simulink model "f_pack"  (R2016b)
settings: Solver=FixedStepDiscrete  StartTime=0.0  StopTime=800000  RelTol=1e-3
undefined symbols (not defined in the file): fft_stages
libraries: xbsIndex_r4 x729, simulink x1, casper_library_misc x1
(part 1 of 6)
settings Model: Creator=andrew  LastModifiedBy=andrew
settings DataIOCC: LimitDataPoints=on  SaveFormat=Array
settings OptimizationCC: ExpressionDepthLimit=2147483647  LifeSpan=inf
settings DebuggingCC: UnderspecifiedInitializationDetection=Classic  MergeDetectMultiDrivingBlocksExec=none  SolverPrmCheckMsg=warning  StateNameClashWarn=warning  SFUnexpectedBacktrackingDiag=warning  SFNoUnconditionalDefaultTransitionDiag=warning  SFExecutionAtInitializationDiag=none
settings HardwareCC: ProdBitPerPointer=32  ProdBitPerSizeT=32  ProdBitPerPtrDiffT=32  ProdLargestAtomicFloat=None  ProdIntDivRoundTo=Undefined  ProdEndianess=Unspecified  ProdWordSize=32  ProdHWDeviceType=32-bit Generic
settings ModelReferenceCC: PropagateSignalLabelsOutOfModel=off
settings GRTTargetCC: TargetLangStandard=C89/C90 (ANSI)  GeneratePreprocessorConditionals=Disable all
settings ConfigComp: CovMetricSettings=dw  CovHtmlReporting=on  CovSaveCumulativeToWorkspaceVar=on  CovSaveSingleToWorkspaceVar=on  CovExternalEMLEnable=off

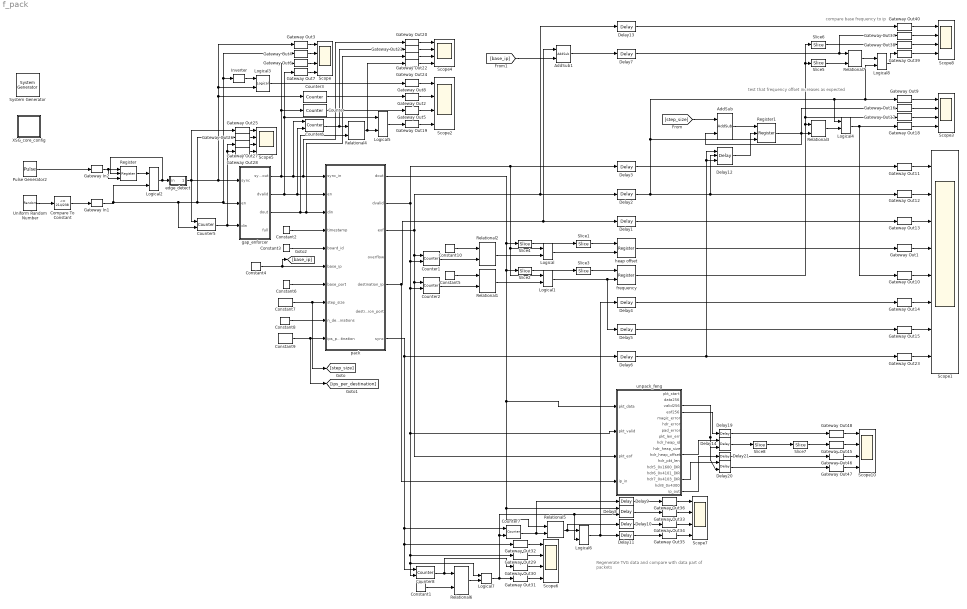
== system f_pack ==
  note: compare base frequency to ip
  note: Regenerate TVG data and compare with data part of
      | packets
  note: test that frequency offset increases as expected
  " System Generator" : xbsIndex_r4/ System Generator  Tag=genX  xilinxfamily=virtex6  part=xc6vsx475t  speed=-1  package=ff1759  synthesis_tool=XST  clock_wrapper=Clock Enables  directory=./r2_128w_32k_16x_r431/sysgen  proj_type=Project Navigator  Synth_file=XST Defaults  Impl_file=ISE Defaults  testbench=off  simulink_period=1  sysclk_period=4.3478  dcm_input_clock_period=100  incr_netlist=off  trim_vbits=Everywhere in SubSystem  dbl_ovrd=According to Block Masks  core_generation=According to Block Masks  run_coregen=off  deprecated_control=off  eval_field=0  block_type=sysgen
      settings: block_version=10.1.3
  AddSub : xbsIndex_r4/AddSub  mode=Addition  use_carryin=off  use_carryout=off  en=off  latency=0  precision=User Defined  arith_type=Unsigned  n_bits=12  bin_pt=0  quantization=Truncate  overflow=Wrap  use_behavioral_HDL=off  hw_selection=Fabric  pipelined=off  dbl_ovrd=off  block_type=addsub
  AddSub1 : xbsIndex_r4/AddSub  mode=Subtraction  use_carryin=off  use_carryout=off  en=off  latency=0  precision=Full  arith_type=Unsigned  n_bits=12  bin_pt=0  quantization=Truncate  overflow=Wrap  use_behavioral_HDL=off  hw_selection=Fabric  pipelined=off  dbl_ovrd=off  block_type=addsub
  Compare To Constant : simulink/Logic and Bit Operations/Compare To Constant  relop=<=  const=214/238  OutDataTypeStr=boolean
  Constant1 : xbsIndex_r4/Constant  const=2  gui_display_data_type=Fixed-point  arith_type=Unsigned  n_bits=6  bin_pt=0  preci_type=Single  exp_width=8  frac_width=24  explicit_period=on  period=1  equ=P=C  opselect=C  inp2=PCIN>>17  opr=+  inp1=P  carry=CIN  dbl_ovrd=off  block_type=constant
  Constant10 : xbsIndex_r4/Constant  const=0  gui_display_data_type=Fixed-point  arith_type=Unsigned  n_bits=10  bin_pt=0  preci_type=Single  exp_width=8  frac_width=24  explicit_period=off  period=1  equ=P=C  opselect=C  inp2=PCIN>>17  opr=+  inp1=P  carry=CIN  dbl_ovrd=off  block_type=constant
  Constant2 : xbsIndex_r4/Constant  const=0  gui_display_data_type=Fixed-point  arith_type=Unsigned  n_bits=48  bin_pt=0  preci_type=Single  exp_width=8  frac_width=24  explicit_period=on  period=1  equ=P=C  opselect=C  inp2=PCIN>>17  opr=+  inp1=P  carry=CIN  dbl_ovrd=off  block_type=constant
  Constant3 : xbsIndex_r4/Constant  const=0  gui_display_data_type=Fixed-point  arith_type=Unsigned  n_bits=16  bin_pt=0  preci_type=Single  exp_width=8  frac_width=24  explicit_period=on  period=1  equ=P=C  opselect=C  inp2=PCIN>>17  opr=+  inp1=P  carry=CIN  dbl_ovrd=off  block_type=constant
  Constant4 : xbsIndex_r4/Constant  const=0  gui_display_data_type=Fixed-point  arith_type=Unsigned  n_bits=32  bin_pt=0  preci_type=Single  exp_width=8  frac_width=24  explicit_period=on  period=1  equ=P=C  opselect=C  inp2=PCIN>>17  opr=+  inp1=P  carry=CIN  dbl_ovrd=off  block_type=constant
  Constant5 : xbsIndex_r4/Constant  const=1  gui_display_data_type=Fixed-point  arith_type=Unsigned  n_bits=10  bin_pt=0  preci_type=Single  exp_width=8  frac_width=24  explicit_period=off  period=1  equ=P=C  opselect=C  inp2=PCIN>>17  opr=+  inp1=P  carry=CIN  dbl_ovrd=off  block_type=constant
  Constant6 : xbsIndex_r4/Constant  const=0  gui_display_data_type=Fixed-point  arith_type=Unsigned  n_bits=16  bin_pt=0  preci_type=Single  exp_width=8  frac_width=24  explicit_period=on  period=1  equ=P=C  opselect=C  inp2=PCIN>>17  opr=+  inp1=P  carry=CIN  dbl_ovrd=off  block_type=constant
  Constant7 : xbsIndex_r4/Constant  const=256  gui_display_data_type=Fixed-point  arith_type=Unsigned  n_bits=12  bin_pt=0  preci_type=Single  exp_width=8  frac_width=24  explicit_period=on  period=1  equ=P=C  opselect=C  inp2=PCIN>>17  opr=+  inp1=P  carry=CIN  dbl_ovrd=off  block_type=constant
  Constant8 : xbsIndex_r4/Constant  const=16  gui_display_data_type=Fixed-point  arith_type=Unsigned  n_bits=9  bin_pt=0  preci_type=Single  exp_width=8  frac_width=24  explicit_period=on  period=1  equ=P=C  opselect=C  inp2=PCIN>>17  opr=+  inp1=P  carry=CIN  dbl_ovrd=off  block_type=constant
  Constant9 : xbsIndex_r4/Constant  const=1  gui_display_data_type=Fixed-point  arith_type=Unsigned  n_bits=6  bin_pt=4  preci_type=Single  exp_width=8  frac_width=24  explicit_period=on  period=1  equ=P=C  opselect=C  inp2=PCIN>>17  opr=+  inp1=P  carry=CIN  dbl_ovrd=off  block_type=constant
  Counter : xbsIndex_r4/Counter  cnt_type=Free Running  cnt_to=Inf  operation=Up  start_count=0  cnt_by_val=1  arith_type=Unsigned  n_bits=16  bin_pt=0  load_pin=off  rst=off  en=on  explicit_period=on  period=1  use_behavioral_HDL=off  implementation=Fabric  dbl_ovrd=off  block_type=counter
  Counter1 : xbsIndex_r4/Counter  cnt_type=Free Running  cnt_to=2^8+10  operation=Up  start_count=0  cnt_by_val=1  arith_type=Unsigned  n_bits=10  bin_pt=0  load_pin=off  rst=on  en=on  explicit_period=on  period=1  use_behavioral_HDL=off  implementation=Fabric  dbl_ovrd=off  block_type=counter
  Counter2 : xbsIndex_r4/Counter  cnt_type=Free Running  cnt_to=2^8+10  operation=Up  start_count=0  cnt_by_val=1  arith_type=Unsigned  n_bits=10  bin_pt=0  load_pin=off  rst=on  en=on  explicit_period=on  period=1  use_behavioral_HDL=off  implementation=Fabric  dbl_ovrd=off  block_type=counter
  Counter3 : xbsIndex_r4/Counter  cnt_type=Free Running  cnt_to=Inf  operation=Up  start_count=0  cnt_by_val=1  arith_type=Unsigned  n_bits=16  bin_pt=0  load_pin=off  rst=off  en=on  explicit_period=on  period=1  use_behavioral_HDL=off  implementation=Fabric  dbl_ovrd=off  block_type=counter
  Counter5 : xbsIndex_r4/Counter  cnt_type=Free Running  cnt_to=Inf  operation=Up  start_count=0  cnt_by_val=1  arith_type=Unsigned  n_bits=256  bin_pt=0  load_pin=off  rst=on  en=on  explicit_period=on  period=1  use_behavioral_HDL=off  implementation=Fabric  dbl_ovrd=off  block_type=counter
  Counter6 : xbsIndex_r4/Counter  cnt_type=Free Running  cnt_to=Inf  operation=Up  start_count=0  cnt_by_val=1  arith_type=Unsigned  n_bits=256  bin_pt=0  load_pin=off  rst=on  en=on  explicit_period=on  period=1  use_behavioral_HDL=off  implementation=Fabric  dbl_ovrd=off  block_type=counter
  Counter7 : xbsIndex_r4/Counter  cnt_type=Free Running  cnt_to=Inf  operation=Up  start_count=0  cnt_by_val=1  arith_type=Unsigned  n_bits=256  bin_pt=0  load_pin=off  rst=on  en=on  explicit_period=on  period=1  use_behavioral_HDL=off  implementation=Fabric  dbl_ovrd=off  block_type=counter
  Counter8 : xbsIndex_r4/Counter  cnt_type=Count Limited  cnt_to=34  operation=Up  start_count=0  cnt_by_val=1  arith_type=Unsigned  n_bits=6  bin_pt=0  load_pin=off  rst=on  en=on  explicit_period=on  period=1  use_behavioral_HDL=off  implementation=Fabric  dbl_ovrd=off  block_type=counter
  Delay{1..7,9..11,13,19,21} (13 alike) : xbsIndex_r4/Delay  rst=off  infoeditControl=Selection of Reset will increase slice count due to use of real FFs and instead of SRLs  en=off  latency=1  reg_retiming=off  dbl_ovrd=off  block_type=delay
  Delay12 : xbsIndex_r4/Delay  rst=on  infoeditControl=Selection of Reset will increase slice count due to use of real FFs and instead of SRLs  en=on  latency=1  reg_retiming=off  dbl_ovrd=off  block_type=delay
      settings: infoedit=Hardware notes: A delay line is a chain, each link of which is an SRL16 or SRL32 followed by a flip-flop.
  Delay14 : xbsIndex_r4/Delay  rst=off  infoeditControl=Selection of Reset will increase slice count due to use of real FFs and instead of SRLs  en=on  latency=1  reg_retiming=off  dbl_ovrd=off  block_type=delay
      settings: infoedit=Hardware notes: A delay line is a chain, each link of which is an SRL16 or SRL32 followed by a flip-flop.
  Delay20 : xbsIndex_r4/Delay  rst=off  infoeditControl=Selection of Reset will increase slice count due to use of real FFs and instead of SRLs  en=on  latency=1  reg_retiming=off  dbl_ovrd=off  block_type=delay
      settings: infoedit=Hardware notes: A delay line is a chain, each link of which is an SRL16 or SRL32 followed by a flip-flop.
  Delay8 : xbsIndex_r4/Delay  rst=off  infoeditControl=Selection of Reset will increase slice count due to use of real FFs and instead of SRLs  en=on  latency=1  reg_retiming=off  dbl_ovrd=off  block_type=delay
      settings: infoedit=Hardware notes: A delay line is a chain, each link of which is an SRL16 or SRL32 followed by a flip-flop.
  Gateway In1 : xbsIndex_r4/Gateway In  gui_display_data_type=Boolean  arith_type=Boolean  n_bits=16  bin_pt=14  preci_type=Single  exp_width=8  frac_width=24  rows=1  columns=1  quantization="Round  (unbiased: +/- Inf)"  overflow=Saturate  period=1  UseAsADC=off  ADCChannel='1'  interface=None  automatic_assignment=on  address_offset=hex2dec('00')  intf_name=''  intf_description=''  default_value=0  timing_constraint=None  locs_specified=off  LOCs={}  io_standard={}  inherit_from_input=off  hdl_port=on  dbl_ovrd=off  block_type=gatewayin
  Gateway In2 : xbsIndex_r4/Gateway In  gui_display_data_type=Boolean  arith_type=Boolean  n_bits=16  bin_pt=14  preci_type=Single  exp_width=8  frac_width=24  rows=1  columns=1  quantization="Round  (unbiased: +/- Inf)"  overflow=Saturate  period=1  UseAsADC=off  ADCChannel='1'  interface=None  automatic_assignment=on  address_offset=hex2dec('00')  intf_name=''  intf_description=''  default_value=0  timing_constraint=None  locs_specified=off  LOCs={}  io_standard={}  inherit_from_input=off  hdl_port=on  dbl_ovrd=off  block_type=gatewayin
  Gateway Out{1..40,45..48} (44 alike) : xbsIndex_r4/Gateway Out  inherit_from_input=off  hdl_port=on  rows=1  columns=1  UseAsDAC=off  DACChannel='1'  interface=None  automatic_assignment=on  address_offset=hex2dec('00')  intf_name=''  intf_description=''  timing_constraint=None  locs_specified=off  LOCs={}  io_standard={}  block_type=gatewayout
  Inverter : xbsIndex_r4/Inverter  en=off  latency=0  dbl_ovrd=off  block_type=inv
  Logical{,1..8} (9 alike) : xbsIndex_r4/Logical  logical_function=AND  inputs=2  en=off  latency=0  precision=Full  arith_type=Unsigned  n_bits=16  bin_pt=0  align_bp=on  dbl_ovrd=off  block_type=logical
  Pulse Generator2 : DiscretePulseGenerator  Period=2^(10+8)  PhaseDelay=2001
  Register : xbsIndex_r4/Register  init=0  rst=on  en=on  dbl_ovrd=off  block_type=register
  Register1 : xbsIndex_r4/Register  init=0  rst=on  en=on  dbl_ovrd=off  block_type=register
  Relational1 : xbsIndex_r4/Relational  mode=a=b  op_type=Bool  en=off  latency=0  dbl_ovrd=off  block_type=relational
  Relational2 : xbsIndex_r4/Relational  mode=a=b  op_type=Bool  en=off  latency=0  dbl_ovrd=off  block_type=relational
  Relational{3..5,7} (4 alike) : xbsIndex_r4/Relational  mode=a!=b  op_type=Bool  en=off  latency=0  dbl_ovrd=off  block_type=relational
  Relational6 : xbsIndex_r4/Relational  mode=a>b  op_type=Bool  en=off  latency=0  dbl_ovrd=off  block_type=relational
  Scope{,2..8,10} (9 alike) : Scope  NumInputPorts=4
  Scope1 : Scope  NumInputPorts=8
  Slice1 : xbsIndex_r4/Slice  nbits=30  boolean_output=off  mode=Two Bit Locations  bit1=0  base1=MSB of Input  bit0=10  base0=LSB of Input  dbl_ovrd=off  block_type=slice
  Slice2 : xbsIndex_r4/Slice  nbits=48  boolean_output=off  mode=Lower Bit Location + Width  bit1=0  base1=MSB of Input  bit0=0  base0=LSB of Input  dbl_ovrd=off  block_type=slice
  Slice3 : xbsIndex_r4/Slice  nbits=12  boolean_output=off  mode=Lower Bit Location + Width  bit1=0  base1=MSB of Input  bit0=0  base0=LSB of Input  dbl_ovrd=off  block_type=slice
  Slice4 : xbsIndex_r4/Slice  nbits=48  boolean_output=off  mode=Lower Bit Location + Width  bit1=0  base1=MSB of Input  bit0=0  base0=LSB of Input  dbl_ovrd=off  block_type=slice
  Slice5 : xbsIndex_r4/Slice  nbits=30  boolean_output=off  mode=Two Bit Locations  bit1=0  base1=MSB of Input  bit0=8  base0=LSB of Input  dbl_ovrd=off  block_type=slice
  Slice6 : xbsIndex_r4/Slice  nbits=30  boolean_output=off  mode=Two Bit Locations  bit1=0  base1=MSB of Input  bit0=8  base0=LSB of Input  dbl_ovrd=off  block_type=slice
  Slice7 : xbsIndex_r4/Slice  nbits=30  boolean_output=off  mode=Two Bit Locations  bit1=0  base1=MSB of Input  bit0=10  base0=LSB of Input  dbl_ovrd=off  block_type=slice
  Slice8 : xbsIndex_r4/Slice  nbits=48  boolean_output=off  mode=Lower Bit Location + Width  bit1=0  base1=MSB of Input  bit0=0  base0=LSB of Input  dbl_ovrd=off  block_type=slice
  Uniform Random Number : UniformRandomNumber  Minimum=0  SampleTime=1
  XSG_core_config : Subsystem  Tag=xps:xsg  AncestorBlock=xps_library/XSG_core_config  mask(xsg core config){hw_sys=SKARAB:xc7vx690t, clk_src=sys_clk, clk_rate=230, sample_period=1, synthesis_tool=XST}
      mask prompts: hw_sys "Hardware Platform"; clk_src "User IP Clock source"; clk_rate "User IP Clock Rate (MHz)"; sample_period "Sample Period"; synthesis_tool "Synthesis Tool:"
      mask help:
      | The XSG Core Config block is used to configure the System Generator design
      | for the casper_xps toolflow. Settings here are used to configure the
      | Xilinx System Generator block parameters automatically, and control toolflow
      | script  execution. It needs to be at the top level of all designs being compiled
      | with the casper_xps toolflow.
      mask init:
      | xps_xsg_conf_mask;
      mask Help: eval('xlWeb([getenv(''MLIB_ROOT''), ''\doc\html\sys_xsg_core_config\sys_xsg_core_config.html''])')
      mask TypeOptions hw_sys: ROACH:sx95t | ROACH:lx110t | ROACH2:sx475t | SNAP:xc7k160t | KC705:xc7k325t | SKARAB:xc7vx690t
      mask Callback hw_sys: xps_xsg_conf_callback
      mask TypeOptions clk_src: sys_clk | aux_clk
      mask Callback clk_src: xps_xsg_conf_callback
      mask Callback clk_rate: xps_xsg_conf_callback
      mask TypeOptions synthesis_tool: Leonardo Spectrum | Synplify | Synplify Pro | XST
      mask Display: fprintf(['MSSGE\n', hw_sys]);
  edge_detect : Subsystem  AncestorBlock=casper_library_misc/edge_detect  mask(edge_detect){edge=Rising, polarity=Active High, x_in=[0 0.08 0.08 0.16 0.16 0.24 0.24 0.32 0.32 0.4], y_in=[-1 -1  1  1  1  1  1  1  1  1], x_out=[0.6 0.68 0.68 0.76 0.76 0.84 0.84 0.92 0.92 1], y_out=[-1 -1  1  1 -1 -1 -1 -1 -1 -1]}
      mask prompts: edge "Edge Type"; polarity "Output Polarity"; x_in "Input X Positions"; y_in "Input Y Positions"; x_out "Output X Positions"; y_out "Output Y Positions"
      mask help: Output is active for one-cycle after each edge of the specified type (i.e. rising, falling or both).
      mask init:
      | edge_detect_init(gcb,...
      |     'edge',edge,...
      |     'polarity',polarity,...
      |     'x_in',x_in,...
      |     'x_out',x_out,...
      |     'y_in',y_in,...
      |     'y_out',y_out);
      | 
      | x_in_num=str2num(getfield(getfield(get_param(gcb,'UserData'),'parameters'),'x_in'));
      | x_out_num=str2num(getfield(getfield(get_param(gcb,'UserData'),'parameters'),'x_out'));
      | y_in_num=str2num(getfield(getfield(get_param(gcb,'UserData'),'parameters'),'y_in'));
      | y_out_num=str2num(getfield(getfield(get_param(gcb,'UserData'),'parameters'),'y_out'));
      settings: AttributesFormatString=|
      | rising edges
      | active high
      mask Help: Output is active for one-cycle after each edge of the specified type (i.e. rising, falling, or both).  Latency is zero.
      mask TypeOptions edge: Rising | Falling | Both
      mask TypeOptions polarity: Active High | Active Low
      mask Display:
      | plot(x_in_num,0.5+y_in_num*0.2);
      | plot(x_out_num,0.5+y_out_num*0.2);
  frequency : xbsIndex_r4/Register  init=0  rst=off  en=on  dbl_ovrd=off  block_type=register
  gap_enforcer : Subsystem  mask{block_size=2^(8+2-5), gap_size=3}
      mask prompts: block_size "data block size"; gap_size "gap size"
  heap offset : xbsIndex_r4/Register  init=0  rst=off  en=on  dbl_ovrd=off  block_type=register
  pack : Subsystem  mask{n_bits_vector=fft_stages-1, n_bits_inputs=3, n_bits_bytes=2, n_bits_packet=8, n_bits_destinations=9, n_bits_ants=8}
      mask prompts: n_bits_vector "total vector length (2^?)"; n_bits_inputs "number of parallel words (2^?)"; n_bits_bytes "bytes per word (2^?)"; n_bits_packet "packet size (2^? words)"; n_bits_destinations "max number destinations (2^?)"; n_bits_ants "max number antennas (2^?)"
  unpack_feng : Subsystem  Tag=casper:spead_unpack  AncestorBlock=casper_library_communications/spead_unpack  mask(spead_unpack_mask){max_pkt_len_bits=10, header_ids=0x1600, 0x4101, 0x4103, header_ind_ids=0x4300, spead_msw=64, spead_lsw=48, spead_version=4, combine_errors=on}
      mask prompts: max_pkt_len_bits "Max pkt length, 2^? 64-bit words"; header_ids "SPEAD direct header IDs (decimal)"; header_ind_ids "SPEAD indirect address IDs (decimal)"; spead_msw "SPEAD Flavour (MSw)"; spead_lsw "SPEAD Flavour (LSw)"; spead_version "SPEAD version"; combine_errors "Combine error flags"
      mask help: This block receives a 64-bit-word stream that contains a SPEAD stream. It checks the SPEAD headers are being correctly received. It presents the user with all headers on the first valid cycle of data along with a flag to indicate a header or packet-length error.
      mask init:
      | %spead_unpack_init(gcb)
  wires:
  Constant2/1 -> pack/4(timestamp)
  Constant3/1 -> pack/5(board_id)
  Constant4/1 -> pack/6(base_ip), [base_ip]
  Constant6/1 -> pack/7(base_port)
  Gateway Out3/1 -> Scope/1
  Gateway Out4/1 -> Scope/2
  Compare To Constant/1 -> Gateway In1/1
  Counter5/1 -> Gateway Out28/1, Gateway Out27/1, gap_enforcer/3(din)
  gap_enforcer/1(sync_out) -> Gateway Out6/1, Counter/1, pack/1(sync_in), Gateway Out20/1, Counter6/1
  gap_enforcer/2(dvalid) -> pack/2(en), Counter6/2, Gateway Out7/1, Logical5/1
  gap_enforcer/3(dout) -> Relational4/2, pack/3(din), Gateway Out22/1
  Gateway Out6/1 -> Scope/3
  Gateway Out7/1 -> Scope/4
  Gateway In1/1 -> Logical2/2, Gateway Out26/1, Inverter/1, Gateway Out4/1, gap_enforcer/2(en), Counter5/2
  Pulse Generator2/1 -> Gateway In2/1
  Gateway Out11/1 -> Scope1/1
  Gateway Out13/1 -> Scope1/3
  Counter2/1 -> Relational1/2
  Constant5/1 -> Relational1/1
  Gateway Out12/1 -> Scope1/2
  Gateway Out10/1 -> Scope1/5
  pack/2(dvalid) -> Counter2/2, Logical7/1, Counter8/2, Gateway Out29/1, unpack_feng/2(pkt_valid), Counter1/2, Delay3/1, Logical1/1, Logical/1
  pack/3(eof) -> unpack_feng/3(pkt_eof), Counter2/1, Counter1/1, Delay13/1, Delay2/1
  Gateway Out14/1 -> Scope1/6
  pack/1(dout) -> Slice2/1, Delay8/1, Relational5/1, unpack_feng/1(pkt_data), Slice4/1
  Gateway Out15/1 -> Scope1/7
  Gateway Out23/1 -> Scope1/8
  Slice3/1 -> frequency/1
  Delay1/1 -> Gateway Out13/1
  Delay3/1 -> Gateway Out11/1
  Delay4/1 -> Gateway Out14/1
  Delay5/1 -> Gateway Out15/1
  Delay6/1 -> Gateway Out23/1, Delay12/1, Delay12/3
  Uniform Random Number/1 -> Compare To Constant/1
  Constant7/1 -> pack/8(step_size), [step_size]
  Constant9/1 -> pack/10(ips_per_destination), [ips_per_destination]
  Constant8/1 -> pack/9(n_destinations)
  Counter1/1 -> Relational2/2
  Constant10/1 -> Relational2/1
  heap offset/1 -> Gateway Out1/1
  Gateway Out1/1 -> Scope1/4
  Slice1/1 -> heap offset/1
  Slice4/1 -> Slice1/1
  Slice2/1 -> Slice3/1
  Logical/1 -> heap offset/2
  Relational2/1 -> Logical/2
  Relational1/1 -> Logical1/2
  Logical1/1 -> Delay5/1, frequency/2
  pack/7(sync) -> Counter7/1, Counter8/1, Gateway Out32/1, Delay6/1
  Gateway In2/1 -> Register/3, Register/1
  Logical2/1 -> Register/2, edge_detect/1(in)
  Counter3/1 -> Gateway Out2/1
  Counter/1 -> Gateway Out5/1
  Gateway Out2/1 -> Scope2/2
  Gateway Out5/1 -> Scope2/3
  Inverter/1 -> Logical3/1
  Gateway Out8/1 -> Scope2/1
  Logical3/1 -> Gateway Out8/1
  edge_detect/1(out) -> Gateway Out25/1, Logical3/2, Gateway Out3/1, Counter3/1, gap_enforcer/1(sync), Counter5/1
  Register/1 -> Logical2/1
  Relational3/1 -> Logical4/2
  Delay2/1 -> Gateway Out12/1, Delay12/2, Logical8/2, Gateway Out9/1, Logical4/1, Register1/3
  Gateway Out9/1 -> Scope3/1
  Gateway Out16/1 -> Scope3/2
  Gateway Out17/1 -> Scope3/3
  Gateway Out18/1 -> Scope3/4
  Logical4/1 -> Gateway Out10/1, Gateway Out18/1
  Counter6/1 -> Gateway Out21/1, Relational4/1
  Relational4/1 -> Gateway Out24/1, Logical5/2
  Gateway Out19/1 -> Scope2/4
  Gateway Out20/1 -> Scope4/1
  Gateway Out21/1 -> Scope4/2
  Gateway Out22/1 -> Scope4/3
  Gateway Out24/1 -> Scope4/4
  Gateway Out25/1 -> Scope5/1
  Gateway Out26/1 -> Scope5/2
  Gateway Out27/1 -> Scope5/3
  Gateway Out28/1 -> Scope5/4
  Logical5/1 -> Gateway Out19/1
  Relational5/1 -> Delay10/1, Logical6/1
  Counter7/1 -> Delay9/1, Relational5/2
  Counter8/1 -> Gateway Out30/1, Relational6/1
  Constant1/1 -> Relational6/2
  Logical6/1 -> Delay4/1, Delay11/1
  Gateway Out32/1 -> Scope6/1
  Gateway Out29/1 -> Scope6/2
  Gateway Out30/1 -> Scope6/3
  Gateway Out31/1 -> Scope6/4
  Gateway Out36/1 -> Scope7/1
  Gateway Out33/1 -> Scope7/2
  Gateway Out34/1 -> Scope7/3
  Gateway Out35/1 -> Scope7/4
  Delay9/1 -> Gateway Out36/1
  Delay8/1 -> Gateway Out33/1
  Delay10/1 -> Gateway Out34/1
  Delay11/1 -> Gateway Out35/1
  Logical7/1 -> Counter7/2, Delay8/2, Logical6/2, Gateway Out31/1
  Relational6/1 -> Logical7/2
  pack/5(destination_ip) -> unpack_feng/4(ip_in), Delay1/1, AddSub1/1
  frequency/1 -> Relational3/1, Slice5/1, Slice6/1, Gateway Out17/1
  [base_ip] -> AddSub1/2
  AddSub1/1 -> Delay7/1
  Relational7/1 -> Logical8/1
  Gateway Out40/1 -> Scope8/1
  Gateway Out37/1 -> Scope8/2
  Gateway Out38/1 -> Scope8/3
  Gateway Out39/1 -> Scope8/4
  Logical8/1 -> Gateway Out39/1
  Slice5/1 -> Relational7/2
  Delay7/1 -> Relational7/1, Gateway Out37/1
  Delay13/1 -> Gateway Out40/1
  Slice6/1 -> Gateway Out38/1
  [step_size] -> AddSub/1
  Delay12/1 -> Register1/2
  AddSub/1 -> Register1/1
  Register1/1 -> Gateway Out16/1, Relational3/2, AddSub/2
  unpack_feng/4(eof256) -> Delay19/1
  unpack_feng/15(hdr7_0x4103_DIR) -> Delay20/1
  unpack_feng/3(valid256) -> Delay20/2, Delay14/2
  Gateway Out48/1 -> Scope10/1
  Gateway Out45/1 -> Scope10/2
  Gateway Out46/1 -> Scope10/3
  Gateway Out47/1 -> Scope10/4
  Delay14/1 -> Slice8/1
  unpack_feng/11(hdr_heap_offset) -> Delay14/1
  Slice8/1 -> Slice7/1
  Delay19/1 -> Gateway Out48/1
  Delay21/1 -> Gateway Out46/1
  Delay20/1 -> Gateway Out47/1
  Slice7/1 -> Gateway Out45/1
  unpack_feng/17(ip_out) -> Delay21/1

== system f_pack/XSG_core_config ==

== system f_pack/edge_detect ==
  in : Inport
  Delay : xbsIndex_r4/Delay  rst=off  infoeditControl=Selection of Reset will increase slice count due to use of real FFs and instead of SRLs  en=off  latency=1  reg_retiming=off  dbl_ovrd=off  block_type=delay
      settings: xl_area=[0, 0, 0, 0, 0, 0, 0]
  Inverter : xbsIndex_r4/Inverter  en=off  latency=0  dbl_ovrd=off  block_type=inv
      settings: xl_area=[0, 0, 0, 0, 0, 0, 0]
  edge_op : xbsIndex_r4/Logical  logical_function=NOR  inputs=2  en=off  latency=0  precision=Full  arith_type=Unsigned  n_bits=8  bin_pt=2  align_bp=on  dbl_ovrd=off  block_type=logical
      settings: xl_area=[0, 0, 0, 0, 0, 0, 0]
  out : Outport
  wires:
  Inverter/1 -> edge_op/1
  edge_op/1 -> out/1
  in/1 -> Inverter/1, Delay/1
  Delay/1 -> edge_op/2

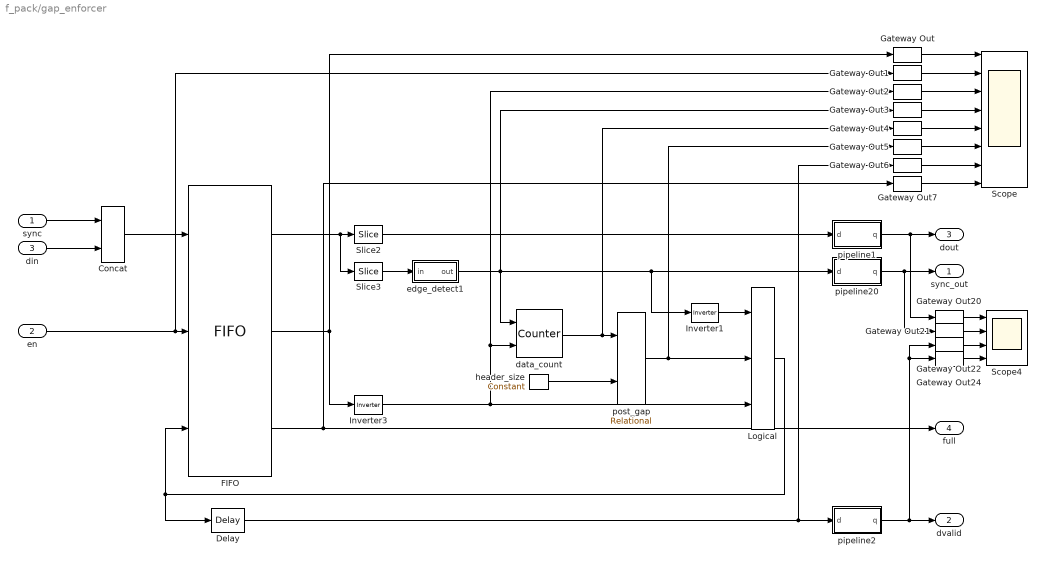
== system f_pack/gap_enforcer ==
  sync : Inport
  en : Inport  Port=2
  din : Inport  Port=3
  Concat : xbsIndex_r4/Concat  num_inputs=2  dbl_ovrd=off  block_type=concat
  Delay : xbsIndex_r4/Delay  rst=off  infoeditControl=Selection of Reset will increase slice count due to use of real FFs and instead of SRLs  en=off  latency=1  reg_retiming=off  dbl_ovrd=off  block_type=delay
  FIFO : xbsIndex_r4/FIFO  mem_type=Distributed RAM  performance_options=Standard_FIFO  embedded_registers=off  depth=64  percent_nbits=1  rst=off  rst_latency=1  en=off  use_dcount=off  use_percent_full_port=off  use_almost_empty=off  almost_empty_thresh=2  use_almost_full=off  almost_full_thresh=14  explicit_period=off  dbl_ovrd=off  block_type=fifo
  Gateway Out{,1..7,20..22,24} (12 alike) : xbsIndex_r4/Gateway Out  inherit_from_input=off  hdl_port=on  rows=1  columns=1  UseAsDAC=off  DACChannel='1'  interface=None  automatic_assignment=on  address_offset=hex2dec('00')  intf_name=''  intf_description=''  timing_constraint=None  locs_specified=off  LOCs={}  io_standard={}  block_type=gatewayout
  Inverter1 : xbsIndex_r4/Inverter  en=off  latency=0  dbl_ovrd=off  block_type=inv
  Inverter3 : xbsIndex_r4/Inverter  en=off  latency=0  dbl_ovrd=off  block_type=inv
  Logical : xbsIndex_r4/Logical  logical_function=AND  inputs=3  en=off  latency=0  precision=Full  arith_type=Unsigned  n_bits=16  bin_pt=0  align_bp=on  dbl_ovrd=off  block_type=logical
  Scope : Scope  NumInputPorts=8
  Scope4 : Scope  NumInputPorts=4
  Slice2 : xbsIndex_r4/Slice  nbits=1  boolean_output=off  mode=Two Bit Locations  bit1=-1  base1=MSB of Input  bit0=0  base0=LSB of Input  dbl_ovrd=off  block_type=slice
  Slice3 : xbsIndex_r4/Slice  nbits=1  boolean_output=on  mode=Upper Bit Location + Width  bit1=0  base1=MSB of Input  bit0=0  base0=LSB of Input  dbl_ovrd=off  block_type=slice
  data_count : xbsIndex_r4/Counter  cnt_type=Count Limited  cnt_to=block_size + gap_size - 1  operation=Up  start_count=0  cnt_by_val=1  arith_type=Unsigned  n_bits=ceil(log2(block_size + gap_size - 1))  bin_pt=0  load_pin=off  rst=on  en=on  explicit_period=on  period=1  use_behavioral_HDL=off  implementation=Fabric  dbl_ovrd=off  block_type=counter
  edge_detect1 : Subsystem  AncestorBlock=casper_library_misc/edge_detect  mask(edge_detect){edge=Rising, polarity=Active High, x_in=[0 0.08 0.08 0.16 0.16 0.24 0.24 0.32 0.32 0.4], y_in=[-1 -1  1  1  1  1  1  1  1  1], x_out=[0.6 0.68 0.68 0.76 0.76 0.84 0.84 0.92 0.92 1], y_out=[-1 -1  1  1 -1 -1 -1 -1 -1 -1]}
      mask prompts: edge "Edge Type"; polarity "Output Polarity"; x_in "Input X Positions"; y_in "Input Y Positions"; x_out "Output X Positions"; y_out "Output Y Positions"
      mask help: Output is active for one-cycle after each edge of the specified type (i.e. rising, falling or both).
      mask init: same as f_pack/edge_detect
      settings: AttributesFormatString=|
      | rising edges
      | active high
      mask Help: Output is active for one-cycle after each edge of the specified type (i.e. rising, falling, or both).  Latency is zero.
      mask TypeOptions edge: Rising | Falling | Both
      mask TypeOptions polarity: Active High | Active Low
      mask Display:
      | plot(x_in_num,0.5+y_in_num*0.2);
      | plot(x_out_num,0.5+y_out_num*0.2);
  header_size : xbsIndex_r4/Constant  const=gap_size-1  gui_display_data_type=Fixed-point  arith_type=Unsigned  n_bits=ceil(log2(block_size+gap_size))  bin_pt=0  preci_type=Single  exp_width=8  frac_width=24  explicit_period=on  period=1  equ=P=C  opselect=C  inp2=PCIN>>17  opr=+  inp1=P  carry=CIN  dbl_ovrd=off  block_type=constant
  pipeline1 : Subsystem  AncestorBlock=casper_library_delays/pipeline  mask(pipeline){latency=2}
      mask help:
      | An explicitly laid-out delay line to avoid mapping to SRL16s
      | for use in pipelining to help achieve timing closure.
      mask init:
      | pipeline_init(gcb,'latency',latency);
      settings: AttributesFormatString=Latency = %<latency>
      mask Display:
      | port_label('input', 1, 'd');
      | port_label('output', 1, 'q');
      | disp(['Z^-', num2str(latency)]);
  pipeline2 : Subsystem  AncestorBlock=casper_library_delays/pipeline  mask(pipeline){latency=2}
      mask help:
      | An explicitly laid-out delay line to avoid mapping to SRL16s
      | for use in pipelining to help achieve timing closure.
      mask init:
      | pipeline_init(gcb,'latency',latency);
      settings: AttributesFormatString=Latency = %<latency>
      mask Display:
      | port_label('input', 1, 'd');
      | port_label('output', 1, 'q');
      | disp(['Z^-', num2str(latency)]);
  pipeline20 : Subsystem  AncestorBlock=casper_library_delays/pipeline  mask(pipeline){latency=2}
      mask help:
      | An explicitly laid-out delay line to avoid mapping to SRL16s
      | for use in pipelining to help achieve timing closure.
      mask init:
      | pipeline_init(gcb,'latency',latency);
      settings: AttributesFormatString=Latency = %<latency>
      mask Display:
      | port_label('input', 1, 'd');
      | port_label('output', 1, 'q');
      | disp(['Z^-', num2str(latency)]);
  post_gap : xbsIndex_r4/Relational  mode=a>b  op_type=Bool  en=off  latency=0  dbl_ovrd=off  block_type=relational
  sync_out : Outport
  dvalid : Outport  Port=2
  dout : Outport  Port=3
  full : Outport  Port=4
  wires:
  edge_detect1/1(out) -> data_count/1, pipeline20/1(d), Inverter1/1, Gateway Out3/1
  post_gap/1 -> Gateway Out5/1, Logical/2
  Slice2/1 -> pipeline1/1(d)
  Slice3/1 -> edge_detect1/1(in)
  FIFO/1 -> Slice3/1, Slice2/1
  Concat/1 -> FIFO/1
  din/1 -> Concat/2
  en/1 -> Gateway Out1/1, FIFO/2
  sync/1 -> Concat/1
  header_size/1 -> post_gap/2
  data_count/1 -> Gateway Out4/1, post_gap/1
  pipeline20/1(q) -> Gateway Out21/1, sync_out/1
  pipeline1/1(q) -> Gateway Out20/1, dout/1
  pipeline2/1(q) -> Gateway Out24/1, Gateway Out22/1, dvalid/1
  Gateway Out4/1 -> Scope/5
  Gateway Out2/1 -> Scope/3
  Gateway Out3/1 -> Scope/4
  Gateway Out/1 -> Scope/1
  Gateway Out1/1 -> Scope/2
  Gateway Out5/1 -> Scope/6
  Gateway Out6/1 -> Scope/7
  Gateway Out7/1 -> Scope/8
  Logical/1 -> Delay/1, FIFO/3
  Delay/1 -> pipeline2/1(d), Gateway Out6/1
  FIFO/3 -> Gateway Out7/1, full/1
  Inverter3/1 -> Logical/3, Gateway Out2/1, data_count/2
  Inverter1/1 -> Logical/1
  FIFO/2 -> Gateway Out/1, Inverter3/1
  Gateway Out20/1 -> Scope4/1
  Gateway Out21/1 -> Scope4/2
  Gateway Out22/1 -> Scope4/3
  Gateway Out24/1 -> Scope4/4
